simulink model "ORC_physical_MathWorks"  (R2017a)
settings: Solver=VariableStepAuto  StartTime=0.0  StopTime=10.0  RelTol=1e-3
undefined symbols (not defined in the file or in its folder): pipe_area, sigbuilder_block
undefined symbols (not defined in the file): boiler_liquid_level, condenser_liquid_level, furnace_temperature, preheat_condenser_liquid_level
libraries: fl_lib x37, nesl_utility x14, RankineCycle_lib x5, simulink x3
(part 2 of 2)

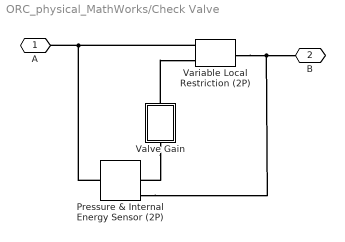
== system ORC_physical_MathWorks/Check Valve ==
  Pressure & Internal Energy Sensor (2P) : fl_lib/Two-Phase Fluid/Sensors/Pressure & Internal Energy Sensor (2P)
      settings: SourceProductName=Foundation Library
  Valve Gain : Subsystem
  Variable Local Restriction (2P) : fl_lib/Two-Phase Fluid/Elements/Variable Local Restriction (2P)  min_area=min_area m^2  max_area=max_area m^2  area=pipe_area m^2  Cd=Cd  B_lam=0.999
      settings: SourceProductName=Foundation Library
  A : PMIOPort  Port=1  Side=Left
  B : PMIOPort  Port=2  Side=Right
  connections:
  Pressure & Internal Energy Sensor (2P)/LConn1 -- Variable Local Restriction (2P)/LConn1 -- A/RConn1
  Variable Local Restriction (2P)/RConn1 -- B/RConn1 -- Pressure & Internal Energy Sensor (2P)/RConn1
  Valve Gain/LConn1 -- Pressure & Internal Energy Sensor (2P)/RConn2
  Valve Gain/RConn1 -- Variable Local Restriction (2P)/LConn2

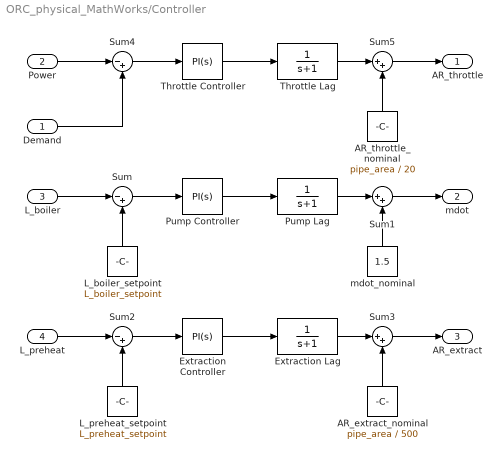
== system ORC_physical_MathWorks/Controller ==
  Demand : Inport
  Power : Inport  Port=2
  L_boiler : Inport  Port=3
  L_preheat : Inport  Port=4
  AR_extract_nominal : Constant  Value=pipe_area / 500
  AR_throttle_nominal : Constant  Value=pipe_area / 20
  Extraction Controller : simulink/Continuous/PID Controller  Controller=PI  TimeDomain=Continuous-time  SampleTime=-1  IntegratorMethod=Forward Euler  FilterMethod=Forward Euler  Form=Ideal  UseFilter=on  ControllerParametersSource=internal  P=-0.01  I=0.01  D=0  N=100  InitialConditionSource=internal  InitialConditionForIntegrator=0  InitialConditionForFilter=0  ExternalReset=none  LimitOutput=on  UpperSaturationLimit=pipe_area * (1/10 - 1/500)  LowerSaturationLimit=- pipe_area / 500  LinearizeAsGain=on  AntiWindupMode=back-calculation  Kb=1  TrackingMode=off  Kt=1  PParamMin=[]  PParamMax=[]  IParamMin=[]  IParamMax=[]  DParamMin=[]  DParamMax=[]  NParamMin=[]  NParamMax=[]  KbParamMin=[]  KbParamMax=[]  KtParamMin=[]  KtParamMax=[]  POutMin=[]  POutMax=[]  IOutMin=[]  IOutMax=[]  DOutMin=[]  DOutMax=[]  NOutMin=[]  NOutMax=[]  KbOutMin=[]  KbOutMax=[]  KtOutMin=[]  KtOutMax=[]  IntegratorOutMin=[]  IntegratorOutMax=[]  FilterOutMin=[]  FilterOutMax=[]  SumOutMin=[]  SumOutMax=[]  SumI1OutMin=[]  SumI1OutMax=[]  SumI2OutMin=[]  SumI2OutMax=[]  SumI3OutMin=[]  SumI3OutMax=[]  SumDOutMin=[]  SumDOutMax=[]  SaturationOutMin=[]  SaturationOutMax=[]  IntegratorContinuousStateAttributes=''  IntegratorStateMustResolveToSignalObject=off  IntegratorRTWStateStorageClass=Auto  FilterContinuousStateAttributes=''  FilterStateMustResolveToSignalObject=off  FilterRTWStateStorageClass=Auto  DifferentiatorICPrevScaledInput=0  DifferentiatorOutMin=[]  DifferentiatorOutMax=[]  InitialConditionSetting=State (most efficient)
  Extraction Lag : TransferFcn  Denominator=[1 1]
  L_boiler_setpoint : Constant  Value=L_boiler_setpoint
  L_preheat_setpoint : Constant  Value=L_preheat_setpoint
  Pump Controller : simulink/Continuous/PID Controller  Controller=PI  TimeDomain=Continuous-time  SampleTime=-1  IntegratorMethod=Forward Euler  FilterMethod=Forward Euler  Form=Ideal  UseFilter=on  ControllerParametersSource=internal  P=50  I=0.01  D=0  N=100  InitialConditionSource=internal  InitialConditionForIntegrator=0  InitialConditionForFilter=0  ExternalReset=none  LimitOutput=on  UpperSaturationLimit=0.5  LowerSaturationLimit=-1.5  LinearizeAsGain=on  AntiWindupMode=back-calculation  Kb=1  TrackingMode=off  Kt=1  PParamMin=[]  PParamMax=[]  IParamMin=[]  IParamMax=[]  DParamMin=[]  DParamMax=[]  NParamMin=[]  NParamMax=[]  KbParamMin=[]  KbParamMax=[]  KtParamMin=[]  KtParamMax=[]  POutMin=[]  POutMax=[]  IOutMin=[]  IOutMax=[]  DOutMin=[]  DOutMax=[]  NOutMin=[]  NOutMax=[]  KbOutMin=[]  KbOutMax=[]  KtOutMin=[]  KtOutMax=[]  IntegratorOutMin=[]  IntegratorOutMax=[]  FilterOutMin=[]  FilterOutMax=[]  SumOutMin=[]  SumOutMax=[]  SumI1OutMin=[]  SumI1OutMax=[]  SumI2OutMin=[]  SumI2OutMax=[]  SumI3OutMin=[]  SumI3OutMax=[]  SumDOutMin=[]  SumDOutMax=[]  SaturationOutMin=[]  SaturationOutMax=[]  IntegratorContinuousStateAttributes=''  IntegratorStateMustResolveToSignalObject=off  IntegratorRTWStateStorageClass=Auto  FilterContinuousStateAttributes=''  FilterStateMustResolveToSignalObject=off  FilterRTWStateStorageClass=Auto  DifferentiatorICPrevScaledInput=0  DifferentiatorOutMin=[]  DifferentiatorOutMax=[]  InitialConditionSetting=State (most efficient)
  Pump Lag : TransferFcn  Denominator=[1 1]
  Sum : Sum  Inputs=|-+
  Sum1 : Sum  Inputs=|++
  Sum2 : Sum  Inputs=|-+
  Sum3 : Sum  Inputs=|++
  Sum4 : Sum  Inputs=|-+
  Sum5 : Sum  Inputs=|++
  Throttle Controller : simulink/Continuous/PID Controller  Controller=PI  TimeDomain=Continuous-time  SampleTime=-1  IntegratorMethod=Forward Euler  FilterMethod=Forward Euler  Form=Ideal  UseFilter=on  ControllerParametersSource=internal  P=1  I=1  D=0  N=100  InitialConditionSource=internal  InitialConditionForIntegrator=0  InitialConditionForFilter=0  ExternalReset=none  LimitOutput=on  UpperSaturationLimit=pipe_area * (1/10 - 1/20)  LowerSaturationLimit=- pipe_area / 20  LinearizeAsGain=on  AntiWindupMode=back-calculation  Kb=1  TrackingMode=off  Kt=1  PParamMin=[]  PParamMax=[]  IParamMin=[]  IParamMax=[]  DParamMin=[]  DParamMax=[]  NParamMin=[]  NParamMax=[]  KbParamMin=[]  KbParamMax=[]  KtParamMin=[]  KtParamMax=[]  POutMin=[]  POutMax=[]  IOutMin=[]  IOutMax=[]  DOutMin=[]  DOutMax=[]  NOutMin=[]  NOutMax=[]  KbOutMin=[]  KbOutMax=[]  KtOutMin=[]  KtOutMax=[]  IntegratorOutMin=[]  IntegratorOutMax=[]  FilterOutMin=[]  FilterOutMax=[]  SumOutMin=[]  SumOutMax=[]  SumI1OutMin=[]  SumI1OutMax=[]  SumI2OutMin=[]  SumI2OutMax=[]  SumI3OutMin=[]  SumI3OutMax=[]  SumDOutMin=[]  SumDOutMax=[]  SaturationOutMin=[]  SaturationOutMax=[]  IntegratorContinuousStateAttributes=''  IntegratorStateMustResolveToSignalObject=off  IntegratorRTWStateStorageClass=Auto  FilterContinuousStateAttributes=''  FilterStateMustResolveToSignalObject=off  FilterRTWStateStorageClass=Auto  DifferentiatorICPrevScaledInput=0  DifferentiatorOutMin=[]  DifferentiatorOutMax=[]  InitialConditionSetting=State (most efficient)
  Throttle Lag : TransferFcn  Denominator=[1 1]
  mdot_nominal : Constant  Value=1.5
  AR_throttle : Outport
  mdot : Outport  Port=2
  AR_extract : Outport  Port=3
  wires:
  L_boiler/1 -> Sum/1
  L_boiler_setpoint/1 -> Sum/2
  Sum/1 -> Pump Controller/1
  mdot_nominal/1 -> Sum1/2
  Pump Controller/1 -> Pump Lag/1
  Sum1/1 -> mdot/1
  Sum3/1 -> AR_extract/1
  L_preheat_setpoint/1 -> Sum2/2
  L_preheat/1 -> Sum2/1
  AR_extract_nominal/1 -> Sum3/2
  Sum5/1 -> AR_throttle/1
  Throttle Controller/1 -> Throttle Lag/1
  Sum4/1 -> Throttle Controller/1
  Power/1 -> Sum4/1
  AR_throttle_nominal/1 -> Sum5/2
  Sum2/1 -> Extraction Controller/1
  Throttle Lag/1 -> Sum5/1
  Pump Lag/1 -> Sum1/1
  Extraction Lag/1 -> Sum3/1
  Extraction Controller/1 -> Extraction Lag/1
  Demand/1 -> Sum4/2

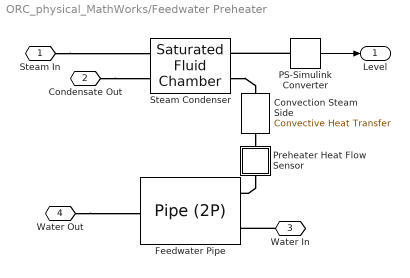
== system ORC_physical_MathWorks/Feedwater Preheater ==
  Convection Steam Side : fl_lib/Thermal/Thermal Elements/Convective Heat Transfer  area=pi * sqrt(4*pipe_area/pi) * pipe_length + fin_area m^2  heat_tr_coeff=steam_heat_coeff W/(m^2 * K)  Q_specify=off  Q_priority=None  Q=0 J/s  Q_nominal_specify=off  Q_nominal_unit=J/s  Q_nominal_value=1  T_specify=off  T_priority=None  T=0 K  T_nominal_specify=off  T_nominal_unit=K  T_nominal_value=1
      settings: SourceProductName=Foundation Library
  Feedwater Pipe : fl_lib/Two-Phase Fluid/Elements/Pipe (2P)  length=pipe_length m  area=pipe_area m^2  Dh=sqrt(4*pipe_area/pi) m  length_add=0.1 * pipe_length m  roughness=15e-6 m  Re_lam=2000  Re_tur=4000  shape_factor=64  Nu_lam=3.66  inertia=0  fluid_spec=1  p_init=p_water_init MPa  T_init=T_water_init degC  x_init=0.2  mdot_init=0 kg/s  time_constant=0.1 s
      settings: SourceProductName=Foundation Library
  PS-Simulink Converter : nesl_utility/PS-Simulink Converter  PhysicalDomain=network_engine_domain  SubClassName=ps_output  LeftPortType=input  RightPortType=output  PseudoPeriodic=off  Frequencies=[]  Unit=1  AffineConversion=off
  Preheater Heat Flow Sensor : Subsystem
  Steam Condenser : RankineCycle_lib/Saturated Fluid Chamber  volume=condenser_volume m^3  area_A=pipe_area m^2  area_B=pipe_area m^2  L_min=0.01  L_max=0.99  p_I_specify=on  p_I_priority=High  p_I=p_steam_init MPa  p_I_nominal_specify=off  p_I_nominal_unit=MPa  p_I_nominal_value=1  L_specify=on  L_priority=High  L=L_init  L_nominal_specify=off  L_nominal_unit=1  L_nominal_value=1
  Steam In : PMIOPort  Port=1  Side=Left
  Condensate Out : PMIOPort  Port=2  Side=Right
  Water In : PMIOPort  Port=3  Side=Right
  Water Out : PMIOPort  Port=4  Side=Left
  Level : Outport
  wires:
  PS-Simulink Converter/1 -> Level/1
  connections:
  Water In/RConn1 -- Feedwater Pipe/LConn1
  Water Out/RConn1 -- Feedwater Pipe/RConn1
  Steam In/RConn1 -- Steam Condenser/LConn1
  Condensate Out/RConn1 -- Steam Condenser/LConn2
  Preheater Heat Flow Sensor/RConn1 -- Feedwater Pipe/LConn2
  PS-Simulink Converter/LConn1 -- Steam Condenser/RConn1
  Convection Steam Side/RConn1 -- Preheater Heat Flow Sensor/LConn1
  Steam Condenser/RConn2 -- Convection Steam Side/LConn1

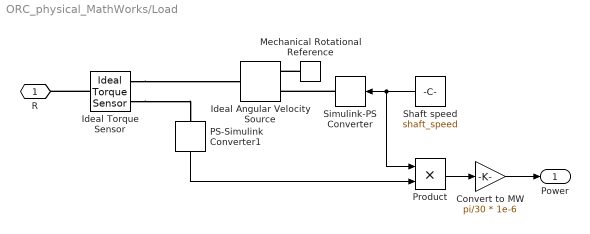
== system ORC_physical_MathWorks/Load ==
  Convert to MW : Gain  Gain=pi/30 * 1e-6
  Ideal Angular Velocity Source : fl_lib/Mechanical/Mechanical Sources/Ideal Angular Velocity Source
      settings: SourceProductName=Foundation Library
  Ideal Torque Sensor : fl_lib/Mechanical/Mechanical Sensors/Ideal Torque Sensor
      settings: SourceProductName=Foundation Library
  Mechanical Rotational Reference : fl_lib/Mechanical/Rotational Elements/Mechanical Rotational Reference
      settings: SourceProductName=Foundation Library
  PS-Simulink Converter1 : nesl_utility/PS-Simulink Converter  PhysicalDomain=network_engine_domain  SubClassName=ps_output  LeftPortType=input  RightPortType=output  PseudoPeriodic=off  Frequencies=[]  Unit=N*m  AffineConversion=off
  Product : Product
  Shaft speed : Constant  Value=shaft_speed
  Simulink-PS Converter : nesl_utility/Simulink-PS Converter  PhysicalDomain=network_engine_domain  SubClassName=ps_input  LeftPortType=input  RightPortType=output  PseudoPeriodic=off  Frequencies=[]  NoiseDistribution=none  NoiseParameters=[]  Unit=rpm  AffineConversion=off  FilteringAndDerivatives=provide  SimscapeFilterOrder=1  InputFilterTimeConstant=0.001  UdotUserProvided=0
  R : PMIOPort  Port=1  Side=Left
  Power : Outport
  wires:
  Product/1 -> Convert to MW/1
  PS-Simulink Converter1/1 -> Product/2
  Shaft speed/1 -> Product/1, Simulink-PS Converter/1
  Convert to MW/1 -> Power/1
  connections:
  Mechanical Rotational Reference/LConn1 -- Ideal Angular Velocity Source/RConn2
  Ideal Torque Sensor/LConn1 -- R/RConn1
  Ideal Torque Sensor/RConn1 -- Ideal Angular Velocity Source/LConn1
  Simulink-PS Converter/RConn1 -- Ideal Angular Velocity Source/RConn1
  Ideal Torque Sensor/RConn2 -- PS-Simulink Converter1/LConn1

== system ORC_physical_MathWorks/Power Demand ==
  Demux : Demux  Tag=STV Demux  Outputs=1
  FromWs : FromWorkspace  Tag=STV FromWs  VariableName=tuvar  SampleTime=0
      SigBuilderData=|
      | common.afterFinalStr = 'Extrapolate'
      | common.sampleTime = 0
      | dataSet.timeRange = [0 100000]
      | dataSet.name = 'Group 1'
      | sbobj.Groups.Name = 'Group 1'
      | sbobj.Groups.Signals.Name = 'Power (MW)'
      | sbobj.Groups.Signals.XData = [0 20000 30000 40000 50000 60000 70000 80000 90000 100000]
      | sbobj.Groups.Signals.YData = [1.15 1.15 1.2 1.2 1.15 1.15 1.1 1.1 1.15 1.15]
      | sbobj.Groups.TimeRange = [0 100000]
  Power (MW) : Outport  Tag=STV Outport
  wires:
  Demux/1 -> Power (MW)/1
  FromWs/1 -> Demux/1

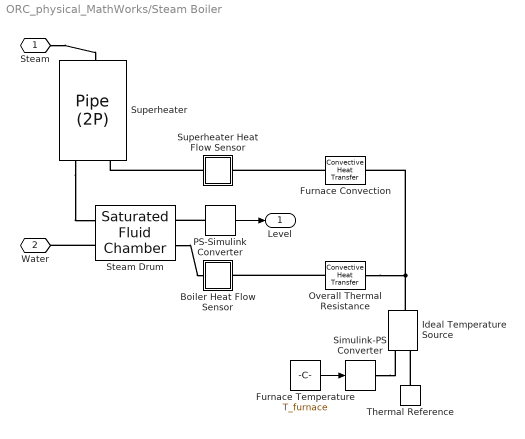
== system ORC_physical_MathWorks/Steam Boiler ==
  Boiler Heat Flow Sensor : Subsystem
  Furnace Convection : fl_lib/Thermal/Thermal Elements/Convective Heat Transfer  area=pi * sqrt(4*pipe_area/pi) * pipe_length + fin_area m^2  heat_tr_coeff=heater_heat_coeff W/(m^2 * K)  Q_specify=off  Q_priority=None  Q=0 J/s  Q_nominal_specify=off  Q_nominal_unit=J/s  Q_nominal_value=1  T_specify=off  T_priority=None  T=0 K  T_nominal_specify=off  T_nominal_unit=K  T_nominal_value=1
      settings: SourceProductName=Foundation Library
  Furnace Temperature : Constant  Value=T_furnace
  Ideal Temperature Source : fl_lib/Thermal/Thermal Sources/Ideal Temperature Source
      settings: SourceProductName=Foundation Library
  Overall Thermal Resistance : fl_lib/Thermal/Thermal Elements/Convective Heat Transfer  area=boiler_area m^2  heat_tr_coeff=boiler_heat_coeff W/(m^2 * K)  Q_specify=off  Q_priority=None  Q=0 J/s  Q_nominal_specify=off  Q_nominal_unit=J/s  Q_nominal_value=1  T_specify=off  T_priority=None  T=0 K  T_nominal_specify=off  T_nominal_unit=K  T_nominal_value=1
      settings: SourceProductName=Foundation Library
  PS-Simulink Converter : nesl_utility/PS-Simulink Converter  PhysicalDomain=network_engine_domain  SubClassName=ps_output  LeftPortType=input  RightPortType=output  PseudoPeriodic=off  Frequencies=[]  Unit=1  AffineConversion=off
  Simulink-PS Converter : nesl_utility/Simulink-PS Converter  PhysicalDomain=network_engine_domain  SubClassName=ps_input  LeftPortType=input  RightPortType=output  PseudoPeriodic=off  Frequencies=[]  NoiseDistribution=none  NoiseParameters=[]  Unit=degC  AffineConversion=on  FilteringAndDerivatives=provide  SimscapeFilterOrder=1  InputFilterTimeConstant=0.001  UdotUserProvided=0
  Steam Drum : RankineCycle_lib/Saturated Fluid Chamber  volume=boiler_volume m^3  area_A=pipe_area m^2  area_B=pipe_area m^2  L_min=0.01  L_max=0.99  p_I_specify=on  p_I_priority=High  p_I=p_init MPa  p_I_nominal_specify=off  p_I_nominal_unit=MPa  p_I_nominal_value=1  L_specify=on  L_priority=High  L=L_init  L_nominal_specify=off  L_nominal_unit=1  L_nominal_value=1
  Superheater : fl_lib/Two-Phase Fluid/Elements/Pipe (2P)  length=pipe_length m  area=pipe_area m^2  Dh=sqrt(4*pipe_area/pi) m  length_add=0.1 * pipe_length m  roughness=15e-6 m  Re_lam=2000  Re_tur=4000  shape_factor=64  Nu_lam=3.66  inertia=0  fluid_spec=3  p_init=p_init MPa  T_init=T_init degC  x_init=0.2  mdot_init=0 kg/s  time_constant=0.1 s
      settings: SourceProductName=Foundation Library
  Superheater Heat Flow Sensor : Subsystem
  Thermal Reference : fl_lib/Thermal/Thermal Elements/Thermal Reference
      settings: SourceProductName=Foundation Library
  Steam : PMIOPort  Port=1  Side=Left
  Water : PMIOPort  Port=2  Side=Left
  Level : Outport
  wires:
  Furnace Temperature/1 -> Simulink-PS Converter/1
  PS-Simulink Converter/1 -> Level/1
  connections:
  Thermal Reference/LConn1 -- Ideal Temperature Source/RConn2
  Steam Drum/LConn2 -- Water/RConn1
  PS-Simulink Converter/LConn1 -- Steam Drum/RConn1
  Ideal Temperature Source/LConn1 -- Overall Thermal Resistance/LConn1 -- Furnace Convection/LConn1
  Overall Thermal Resistance/RConn1 -- Boiler Heat Flow Sensor/LConn1
  Furnace Convection/RConn1 -- Superheater Heat Flow Sensor/LConn1
  Simulink-PS Converter/RConn1 -- Ideal Temperature Source/RConn1
  Steam Drum/RConn2 -- Boiler Heat Flow Sensor/RConn1
  Superheater Heat Flow Sensor/RConn1 -- Superheater/LConn2
  Steam/RConn1 -- Superheater/RConn1
  Superheater/LConn1 -- Steam Drum/LConn1

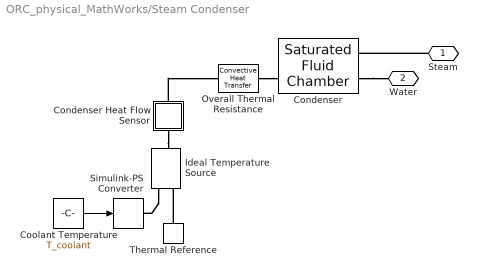
== system ORC_physical_MathWorks/Steam Condenser ==
  Condenser : RankineCycle_lib/Saturated Fluid Chamber  volume=condenser_volume m^3  area_A=pipe_area m^2  area_B=pipe_area m^2  L_min=0.01  L_max=0.99  p_I_specify=on  p_I_priority=High  p_I=p_init MPa  p_I_nominal_specify=off  p_I_nominal_unit=MPa  p_I_nominal_value=1  L_specify=on  L_priority=High  L=L_init  L_nominal_specify=off  L_nominal_unit=1  L_nominal_value=1
  Condenser Heat Flow Sensor : Subsystem
  Coolant Temperature : Constant  Value=T_coolant
  Ideal Temperature Source : fl_lib/Thermal/Thermal Sources/Ideal Temperature Source
      settings: SourceProductName=Foundation Library
  Overall Thermal Resistance : fl_lib/Thermal/Thermal Elements/Convective Heat Transfer  area=condenser_area m^2  heat_tr_coeff=condenser_heat_coeff W/(m^2 * K)  Q_specify=off  Q_priority=None  Q=0 J/s  Q_nominal_specify=off  Q_nominal_unit=J/s  Q_nominal_value=1  T_specify=off  T_priority=None  T=0 K  T_nominal_specify=off  T_nominal_unit=K  T_nominal_value=1
      settings: SourceProductName=Foundation Library
  Simulink-PS Converter : nesl_utility/Simulink-PS Converter  PhysicalDomain=network_engine_domain  SubClassName=ps_input  LeftPortType=input  RightPortType=output  PseudoPeriodic=off  Frequencies=[]  NoiseDistribution=none  NoiseParameters=[]  Unit=degC  AffineConversion=on  FilteringAndDerivatives=provide  SimscapeFilterOrder=1  InputFilterTimeConstant=0.001  UdotUserProvided=0
  Thermal Reference : fl_lib/Thermal/Thermal Elements/Thermal Reference
      settings: SourceProductName=Foundation Library
  Steam : PMIOPort  Port=1  Side=Right
  Water : PMIOPort  Port=2  Side=Right
  wires:
  Coolant Temperature/1 -> Simulink-PS Converter/1
  connections:
  Overall Thermal Resistance/RConn1 -- Condenser/RConn2
  Condenser/LConn2 -- Water/RConn1
  Thermal Reference/LConn1 -- Ideal Temperature Source/RConn2
  Steam/RConn1 -- Condenser/LConn1
  Ideal Temperature Source/RConn1 -- Simulink-PS Converter/RConn1
  Condenser Heat Flow Sensor/RConn1 -- Ideal Temperature Source/LConn1
  Condenser Heat Flow Sensor/LConn1 -- Overall Thermal Resistance/LConn1

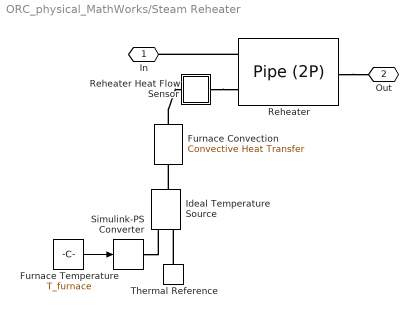
== system ORC_physical_MathWorks/Steam Reheater ==
  Furnace Convection : fl_lib/Thermal/Thermal Elements/Convective Heat Transfer  area=pi * sqrt(4*pipe_area/pi) * pipe_length + fin_area m^2  heat_tr_coeff=heater_heat_coeff W/(m^2 * K)  Q_specify=off  Q_priority=None  Q=0 J/s  Q_nominal_specify=off  Q_nominal_unit=J/s  Q_nominal_value=1  T_specify=off  T_priority=None  T=0 K  T_nominal_specify=off  T_nominal_unit=K  T_nominal_value=1
      settings: SourceProductName=Foundation Library
  Furnace Temperature : Constant  Value=T_furnace
  Ideal Temperature Source : fl_lib/Thermal/Thermal Sources/Ideal Temperature Source
      settings: SourceProductName=Foundation Library
  Reheater : fl_lib/Two-Phase Fluid/Elements/Pipe (2P)  length=pipe_length m  area=pipe_area m^2  Dh=sqrt(4*pipe_area/pi) m  length_add=0.1 * pipe_length m  roughness=15e-6 m  Re_lam=2000  Re_tur=4000  shape_factor=64  Nu_lam=3.66  inertia=0  fluid_spec=3  p_init=p_init MPa  T_init=T_init degC  x_init=0.2  mdot_init=0 kg/s  time_constant=0.1 s
      settings: SourceProductName=Foundation Library
  Reheater Heat Flow Sensor : Subsystem
  Simulink-PS Converter : nesl_utility/Simulink-PS Converter  PhysicalDomain=network_engine_domain  SubClassName=ps_input  LeftPortType=input  RightPortType=output  PseudoPeriodic=off  Frequencies=[]  NoiseDistribution=none  NoiseParameters=[]  Unit=degC  AffineConversion=on  FilteringAndDerivatives=provide  SimscapeFilterOrder=1  InputFilterTimeConstant=0.001  UdotUserProvided=0
  Thermal Reference : fl_lib/Thermal/Thermal Elements/Thermal Reference
      settings: SourceProductName=Foundation Library
  In : PMIOPort  Port=1  Side=Left
  Out : PMIOPort  Port=2  Side=Right
  wires:
  Furnace Temperature/1 -> Simulink-PS Converter/1
  connections:
  Reheater/LConn1 -- In/RConn1
  Reheater/RConn1 -- Out/RConn1
  Thermal Reference/LConn1 -- Ideal Temperature Source/RConn2
  Simulink-PS Converter/RConn1 -- Ideal Temperature Source/RConn1
  Ideal Temperature Source/LConn1 -- Furnace Convection/LConn1
  Reheater Heat Flow Sensor/RConn1 -- Reheater/LConn2
  Furnace Convection/RConn1 -- Reheater Heat Flow Sensor/LConn1

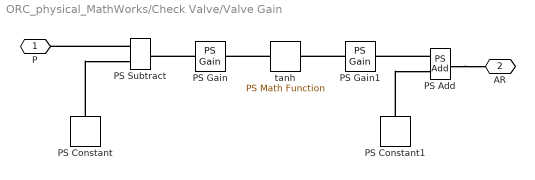
== system ORC_physical_MathWorks/Check Valve/Valve Gain ==
  PS Add : fl_lib/Physical Signals/Functions/PS Add
      settings: SourceProductName=Foundation Library
  PS Constant : fl_lib/Physical Signals/Sources/PS Constant  constant=(max_dp + min_dp) / 2
      settings: SourceProductName=Foundation Library
  PS Constant1 : fl_lib/Physical Signals/Sources/PS Constant  constant=(max_area + min_area) / 2
      settings: SourceProductName=Foundation Library
  PS Gain : fl_lib/Physical Signals/Functions/PS Gain  gain=6 / (max_dp - min_dp)
      settings: SourceProductName=Foundation Library
  PS Gain1 : fl_lib/Physical Signals/Functions/PS Gain  gain=(max_area - min_area) / 2
      settings: SourceProductName=Foundation Library
  PS Subtract : fl_lib/Physical Signals/Functions/PS Subtract
      settings: SourceProductName=Foundation Library
  tanh : fl_lib/Physical Signals/Functions/PS Math Function  fcn_choice=10
      settings: SourceProductName=Foundation Library
  P : PMIOPort  Port=1  Side=Left
  AR : PMIOPort  Port=2  Side=Right
  connections:
  PS Add/LConn1 -- PS Gain1/RConn1
  PS Gain/LConn1 -- PS Subtract/RConn1
  PS Constant/RConn1 -- PS Subtract/LConn2
  PS Constant1/RConn1 -- PS Add/LConn2
  PS Subtract/LConn1 -- P/RConn1
  PS Add/RConn1 -- AR/RConn1
  tanh/LConn1 -- PS Gain/RConn1
  PS Gain1/LConn1 -- tanh/RConn1

== system ORC_physical_MathWorks/Feedwater Preheater/Preheater Heat Flow Sensor ==
  Ideal Heat Flow Sensor : fl_lib/Thermal/Thermal Sensors/Ideal Heat Flow Sensor
      settings: SourceProductName=Foundation Library
  A : PMIOPort  Port=1  Side=Left
  B : PMIOPort  Port=2  Side=Right
  connections:
  Ideal Heat Flow Sensor/RConn2 -- B/RConn1
  Ideal Heat Flow Sensor/LConn1 -- A/RConn1

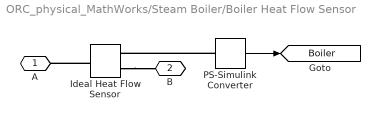
== system ORC_physical_MathWorks/Steam Boiler/Boiler Heat Flow Sensor ==
  Ideal Heat Flow Sensor : fl_lib/Thermal/Thermal Sensors/Ideal Heat Flow Sensor
      settings: SourceProductName=Foundation Library
  PS-Simulink Converter : nesl_utility/PS-Simulink Converter  PhysicalDomain=network_engine_domain  SubClassName=ps_output  LeftPortType=input  RightPortType=output  PseudoPeriodic=off  Frequencies=[]  Unit=MW  AffineConversion=off
  A : PMIOPort  Port=1  Side=Left
  B : PMIOPort  Port=2  Side=Right
  tag scope: Boiler=global
  wires:
  PS-Simulink Converter/1 -> [Boiler]
  connections:
  Ideal Heat Flow Sensor/RConn2 -- B/RConn1
  Ideal Heat Flow Sensor/LConn1 -- A/RConn1
  PS-Simulink Converter/LConn1 -- Ideal Heat Flow Sensor/RConn1

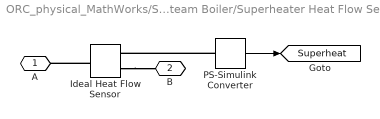
== system ORC_physical_MathWorks/Steam Boiler/Superheater Heat Flow Sensor ==
  Ideal Heat Flow Sensor : fl_lib/Thermal/Thermal Sensors/Ideal Heat Flow Sensor
      settings: SourceProductName=Foundation Library
  PS-Simulink Converter : nesl_utility/PS-Simulink Converter  PhysicalDomain=network_engine_domain  SubClassName=ps_output  LeftPortType=input  RightPortType=output  PseudoPeriodic=off  Frequencies=[]  Unit=MW  AffineConversion=off
  A : PMIOPort  Port=1  Side=Left
  B : PMIOPort  Port=2  Side=Right
  tag scope: Superheat=global
  wires:
  PS-Simulink Converter/1 -> [Superheat]
  connections:
  PS-Simulink Converter/LConn1 -- Ideal Heat Flow Sensor/RConn1
  Ideal Heat Flow Sensor/LConn1 -- A/RConn1
  Ideal Heat Flow Sensor/RConn2 -- B/RConn1

== system ORC_physical_MathWorks/Steam Condenser/Condenser Heat Flow Sensor ==
  Ideal Heat Flow Sensor : fl_lib/Thermal/Thermal Sensors/Ideal Heat Flow Sensor
      settings: SourceProductName=Foundation Library
  A : PMIOPort  Port=1  Side=Left
  B : PMIOPort  Port=2  Side=Right
  connections:
  Ideal Heat Flow Sensor/RConn2 -- B/RConn1
  Ideal Heat Flow Sensor/LConn1 -- A/RConn1

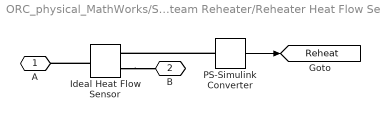
== system ORC_physical_MathWorks/Steam Reheater/Reheater Heat Flow Sensor ==
  Ideal Heat Flow Sensor : fl_lib/Thermal/Thermal Sensors/Ideal Heat Flow Sensor
      settings: SourceProductName=Foundation Library
  PS-Simulink Converter : nesl_utility/PS-Simulink Converter  PhysicalDomain=network_engine_domain  SubClassName=ps_output  LeftPortType=input  RightPortType=output  PseudoPeriodic=off  Frequencies=[]  Unit=MW  AffineConversion=off
  A : PMIOPort  Port=1  Side=Left
  B : PMIOPort  Port=2  Side=Right
  tag scope: Reheat=global
  wires:
  PS-Simulink Converter/1 -> [Reheat]
  connections:
  PS-Simulink Converter/LConn1 -- Ideal Heat Flow Sensor/RConn1
  Ideal Heat Flow Sensor/LConn1 -- A/RConn1
  Ideal Heat Flow Sensor/RConn2 -- B/RConn1
